simulink model "Teste_sem_maquina_sincrona"  (R2016a)
settings: Solver=VariableStepAuto  StartTime=0.0  StopTime=0.01  RelTol=1e-3
undefined symbols (not defined in the file or in its folder): D1, Delta, Ts
libraries: powerlib x42, simulink x4, simulink_extras x4, electricdrivelib x1, powerlib_meascontrol x1
settings Model: Creator=Joao  LastModifiedBy=Joao

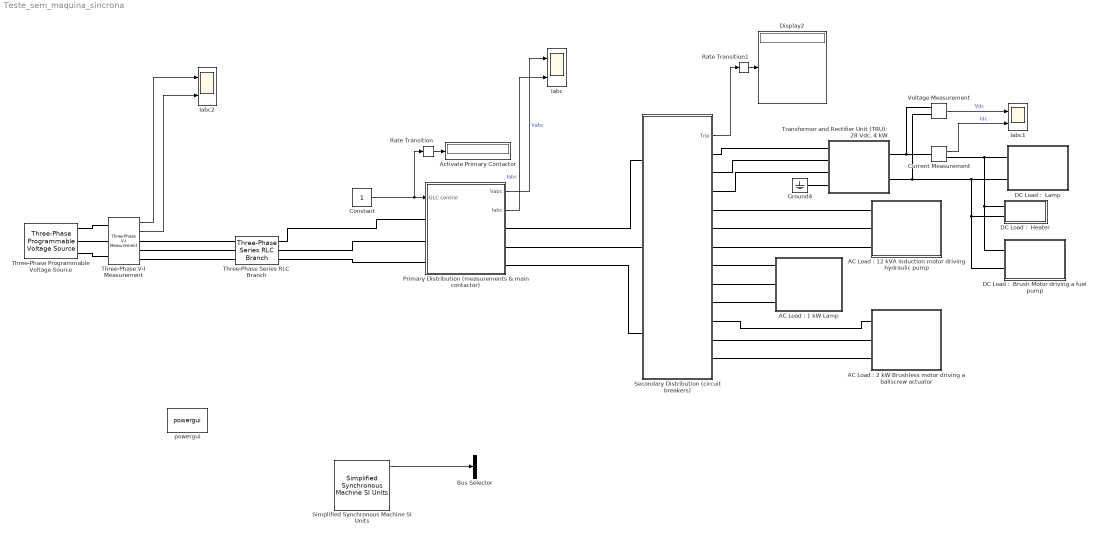
== system Teste_sem_maquina_sincrona ==
  "AC Load : 1 kW Lamp" : Subsystem
      mask Display: image(imread('power_aircraft_distribution_ACLamp.jpg','jpg'))
  "AC Load : 12 kVA induction motor driving hydraulic pump" : Subsystem
      mask Display: image(imread('power_aircraft_distribution_EnginePump.jpg','jpg'))
  "AC Load : 2 kW Brushless motor driving a ballscrew actuator" : Subsystem
      mask Display: image(imread('power_aircraft_distribution_ballscrew.jpg','jpg'))
  Activate Primary Contactor : Display
      settings: SampleTime=1e-2
  Bus Selector : BusSelector  OutputSignals=signal1,signal2
  Constant : Constant
  Current Measurement : powerlib/Measurements/Current Measurement  PhasorSimulation=off  OutputType=Complex  PSBequivalent=0
  "DC Load :  Brush Motor driving a fuel pump" : Subsystem
      mask Display: image(imread('power_aircraft_distribution_FuelPump.jpg','jpg'))
  "DC Load :  Heater" : Subsystem
      mask Display: image(imread('power_aircraft_distribution_heater.jpg','jpg'))
  "DC Load :  Lamp" : Subsystem
      mask Display: image(imread('power_aircraft_distribution_DCLamp.jpg','jpg'))
  Display2 : Display
      settings: SampleTime=1e-2
  Ground4 : powerlib/Elements/Ground  LConnTagsString=a
  Iabc : Scope  NumInputPorts=2
  Iabc1 : Scope  NumInputPorts=2
  Iabc2 : Scope  NumInputPorts=2
  Primary Distribution (measurements & main contactor) : Subsystem
  Rate Transition : RateTransition  OutPortSampleTimeOpt=Inherit  OutPortSampleTime=Ts
  Rate Transition1 : RateTransition  OutPortSampleTimeOpt=Inherit  OutPortSampleTime=Ts
  Secondary Distribution (circuit breakers) : Subsystem  mask{FuseA=25, FuseB=200, FuseC=5, FuseD=30}
      mask prompts: FuseA "Breaker  TRU (Amps RMS)"; FuseB "Breaker AC motor (Amps RMS)"; FuseC "Breaker Lamp (Amps RMS)"; FuseD "Breaker Brushless (Amps RMS)"
  Simplified Synchronous Machine SI Units : powerlib/Machines/Simplified Synchronous Machine SI Units  ConnectionType=3-wire Y  MechanicalLoad=Mechanical power Pm  MeasurementBus=off  NominalParameters=[187e6 13800 60]  Mechanical=[3.895e6 0 20]  InternalRL="[0.0204  0.8104e-3]"  InitialConditions="[ 0,0   0,0,0   0,0,0 ]"  Units=1  LoadFlowParameters=[1,0,0,0,0]  TsPowergui=0  TsBlock=-1  BusType=PV  Pref=0  Qref=0  Qmin=-inf  Qmax=+inf  PLF=0  QLF=0
  Three-Phase Programmable Voltage Source : powerlib/Electrical Sources/Three-Phase Programmable Voltage Source  PositiveSequence="[115*sqrt(3)  0 400]"  VariationEntity=None  VariationType=Table of time-amplitude pairs  VariationTypeAlt=Step  VariationStep=0.5  VariationRate=10  VariationMagnitude=0.3  VariationFrequency=2  VariationTiming=[1 2]  VariationPhaseA=off  Amplitudes=[1 0.8 1.2 1.0]  TimeValues=[0 0.1 0.15 0.2]  HarmonicGeneration=off  HarmonicA=[3 0.2 -25 0]  HarmonicB=[2 0.15 35 2]  Timing="[0.05  3]"  BusType=swing  Pref=0  Qref=0  Qmin=-inf  Qmax=inf
  Three-Phase Series RLC Branch : powerlib/Elements/Three-Phase Series RLC Branch  LConnTagsString=A|B|C  RConnTagsString=A|B|C  BranchType=RL  Resistance=0.2  Inductance=8e-4  Capacitance=0  Measurements=None
  Three-Phase V-I Measurement : powerlib/Measurements/Three-Phase V-I Measurement  VoltageMeasurement=phase-to-ground  SetLabelV=off  LabelV=Vabc  Vpu=off  VpuLL=off  CurrentMeasurement=yes  SetLabelI=off  LabelI=Iabc  Ipu=off  Pbase=100e6  Vbase=500e3  OutputType=Complex  PhasorSimulation=off  PSBequivalent=0
  "Transformer and Rectifier Unit (TRU): 28 Vdc, 4 kW" : Subsystem
      mask Display: image(imread('power_aircraft_distribution_TRU.jpg','jpg'))
  Voltage Measurement : powerlib/Measurements/Voltage Measurement  PhasorSimulation=off  OutputType=Complex  PSBequivalent=0
  powergui : powerlib/powergui  Priority=1  SimulationMode=Discrete  SolverType=Tustin/Backward Euler (TBE)  SampleTime=1e-7  frequency=60  SPID=off  DisableSnubberDevices=off  DisableRonSwitches=off  DisableVfSwitches=off  SwTol=0  DisplayEquations=off  Interpol=off  ExternalGateDelay=off  methode=off  Ts=10  FunctionMessages=off  echomessages=off  HookPort=off  EnableUseOfTLC=off  x0status=blocks  frequencyindice=0  Pbase=100e6  ErrMax=1e-4  Iterations=50  UnitsV=kV  UnitsW=MW  buscounter=0  RestoreLinks=warning  ResistiveCurrentMeasurement=off  Frange=[0:2:500]  Ylog=off  Xlog=on  ShowGrid=off  save=off  variable=ZData  structure=0  ZoomFFT=off  StartTime=0.0  cycles=1  DisplayStyle=1  fundamental=60  FreqAxis=off  MaxFrequency=1000  frequencyindicesteady=1  RmsSteady=1  display=off
  wires:
  Constant/1 -> Rate Transition/1, Primary Distribution (measurements & main contactor)/1(GLC control)
  Secondary Distribution (circuit breakers)/1(Trip) -> Rate Transition1/1
  Current Measurement/1 -> Iabc1/2  "Idc"
  Voltage Measurement/1 -> Iabc1/1  "Vdc"
  Rate Transition/1 -> Activate Primary Contactor/1
  Rate Transition1/1 -> Display2/1
  Three-Phase V-I Measurement/1 -> Iabc2/1
  Three-Phase V-I Measurement/2 -> Iabc2/2
  Primary Distribution (measurements & main contactor)/1(Vabc) -> Iabc/1  "Vabc"
  Primary Distribution (measurements & main contactor)/2(Iabc) -> Iabc/2  "Iabc"
  Simplified Synchronous Machine SI Units/1 -> Bus Selector/1
  connections:
  Current Measurement/RConn1 -- "DC Load :  Lamp"/LConn1 -- "DC Load :  Heater"/LConn1 -- "DC Load :  Brush Motor driving a fuel pump"/LConn1
  Voltage Measurement/LConn1 -- "Transformer and Rectifier Unit (TRU): 28 Vdc, 4 kW"/RConn1 -- Current Measurement/LConn1
  "DC Load :  Lamp"/LConn2 -- Voltage Measurement/LConn2 -- "Transformer and Rectifier Unit (TRU): 28 Vdc, 4 kW"/RConn2 -- "DC Load :  Heater"/LConn2 -- "DC Load :  Brush Motor driving a fuel pump"/LConn2
  Secondary Distribution (circuit breakers)/RConn8 -- "AC Load : 1 kW Lamp"/LConn2
  Secondary Distribution (circuit breakers)/RConn10 -- "AC Load : 2 kW Brushless motor driving a ballscrew actuator"/LConn1
  Secondary Distribution (circuit breakers)/RConn4 -- "AC Load : 12 kVA induction motor driving hydraulic pump"/LConn1
  Secondary Distribution (circuit breakers)/RConn12 -- "AC Load : 2 kW Brushless motor driving a ballscrew actuator"/LConn3
  Secondary Distribution (circuit breakers)/RConn11 -- "AC Load : 2 kW Brushless motor driving a ballscrew actuator"/LConn2
  Ground4/LConn1 -- "Transformer and Rectifier Unit (TRU): 28 Vdc, 4 kW"/LConn4
  Secondary Distribution (circuit breakers)/LConn2 -- Primary Distribution (measurements & main contactor)/RConn2
  Secondary Distribution (circuit breakers)/LConn3 -- Primary Distribution (measurements & main contactor)/RConn3
  Secondary Distribution (circuit breakers)/RConn6 -- "AC Load : 12 kVA induction motor driving hydraulic pump"/LConn3
  Secondary Distribution (circuit breakers)/RConn5 -- "AC Load : 12 kVA induction motor driving hydraulic pump"/LConn2
  Secondary Distribution (circuit breakers)/RConn7 -- "AC Load : 1 kW Lamp"/LConn1
  Secondary Distribution (circuit breakers)/RConn2 -- "Transformer and Rectifier Unit (TRU): 28 Vdc, 4 kW"/LConn2
  Secondary Distribution (circuit breakers)/RConn9 -- "AC Load : 1 kW Lamp"/LConn3
  Secondary Distribution (circuit breakers)/RConn1 -- "Transformer and Rectifier Unit (TRU): 28 Vdc, 4 kW"/LConn1
  Primary Distribution (measurements & main contactor)/RConn1 -- Secondary Distribution (circuit breakers)/LConn1
  Secondary Distribution (circuit breakers)/RConn3 -- "Transformer and Rectifier Unit (TRU): 28 Vdc, 4 kW"/LConn3
  Primary Distribution (measurements & main contactor)/LConn1 -- Three-Phase Series RLC Branch/RConn1
  Primary Distribution (measurements & main contactor)/LConn2 -- Three-Phase Series RLC Branch/RConn2
  Primary Distribution (measurements & main contactor)/LConn3 -- Three-Phase Series RLC Branch/RConn3
  Three-Phase Programmable Voltage Source/RConn1 -- Three-Phase V-I Measurement/LConn1
  Three-Phase Programmable Voltage Source/RConn2 -- Three-Phase V-I Measurement/LConn2
  Three-Phase Programmable Voltage Source/RConn3 -- Three-Phase V-I Measurement/LConn3
  Three-Phase V-I Measurement/RConn1 -- Three-Phase Series RLC Branch/LConn1
  Three-Phase V-I Measurement/RConn2 -- Three-Phase Series RLC Branch/LConn2
  Three-Phase V-I Measurement/RConn3 -- Three-Phase Series RLC Branch/LConn3

== system Teste_sem_maquina_sincrona/AC Load : 1 kW Lamp ==
  note: AC Load
  Lamp 1000 Watts : powerlib/Elements/Three-Phase Series RLC Load  LConnTagsString=A|B|C  Configuration=Y (grounded)  NominalVoltage=200  Vabc=[1e3 1e3 1e3]  Vabcp=[1e3 1e3 1e3]  NominalFrequency=400  UnbalancedPower=off  ActivePower=1000  InductivePower=0  CapacitivePower=0  Pabc=[10e3 9e3 11e3]  QLabc=[100 90 110]  QCabc=[100 90 110]  Pabcp=[10e3 9e3 11e3]  QLabcp=[100 90 110]  QCabcp=[100 90 110]  Measurements=None  LoadType=constant Z
  A : PMIOPort  Port=1  Side=Left
  B : PMIOPort  Port=2  Side=Left
  C : PMIOPort  Port=3  Side=Left
  connections:
  A/RConn1 -- Lamp 1000 Watts/LConn1
  B/RConn1 -- Lamp 1000 Watts/LConn2
  C/RConn1 -- Lamp 1000 Watts/LConn3

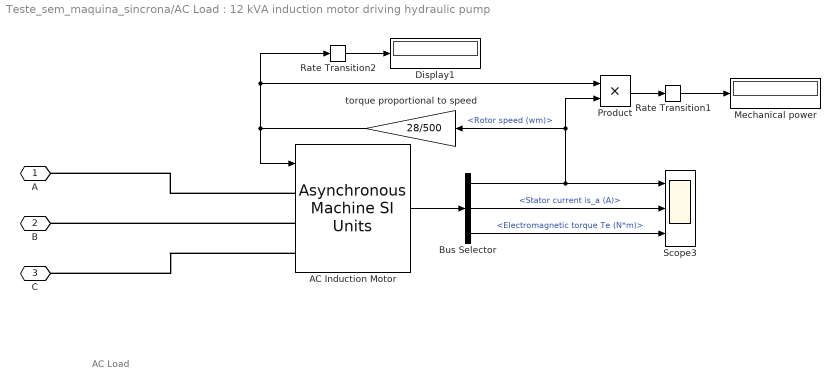
== system Teste_sem_maquina_sincrona/AC Load : 12 kVA induction motor driving hydraulic pump ==
  note: AC Load
  AC Induction Motor : powerlib/Machines/Asynchronous Machine SI Units  RotorType=Squirrel-cage  PresetModel=No  MechanicalLoad=Torque Tm  ShowDetailedParameters=on  ReferenceFrame=Rotor  Units=SI  MeasurementBus=off  NominalParameters=[12e3 200 400]  Stator=[0.2761 0.002191/10]  Rotor=[0.16 0.002191/10]  Cage1=[ 0.022 0.226/377]  Cage2=[ 0.022 0.226/377]  Lm=0.07614  Mechanical=[0.01 0 8]  PolePairs=8  InitialConditions=[1,0 0,0,0 0,0,0]  SimulateSaturation=off  Saturation=[14.03593122, 27.81365428, 53.79336849, 72.68890987, 97.98006896, 148.6815601, 215.7428561, 302.9841135, 428.7778367 ; 230, 322, 414, 460, 506, 552, 598, 644, 690]  LoadFlowParameters=0  TsPowergui=0  TsBlock=-1  IterativeModel=Trapezoidal non iterative  IterativeDiscreteModel=Trapezoidal non iterative  Pmec=0
  Bus Selector : BusSelector  OutputSignals=Mechanical.Rotor speed (wm),Stator measurements.Stator current is_a (A),Mechanical.Electromagnetic torque Te (N*m)
  Display1 : Display
      settings: SampleTime=1e-2
  Mechanical power : Display
      settings: SampleTime=1e-2
  Product : Product  RndMeth=Zero
  Rate Transition1 : RateTransition  OutPortSampleTimeOpt=Inherit  OutPortSampleTime=Ts
  Rate Transition2 : RateTransition  OutPortSampleTimeOpt=Inherit  OutPortSampleTime=Ts
  Scope3 : Scope  NumInputPorts=3
  torque proportional to speed : Gain  Gain=28/500
  A : PMIOPort  Port=1  Side=Left
  B : PMIOPort  Port=2  Side=Left
  C : PMIOPort  Port=3  Side=Left
  wires:
  AC Induction Motor/1 -> Bus Selector/1
  Bus Selector/1 -> Scope3/1, torque proportional to speed/1, Product/2  "<Rotor speed (wm)>"
  torque proportional to speed/1 -> AC Induction Motor/1, Product/1, Rate Transition2/1
  Product/1 -> Rate Transition1/1
  Bus Selector/2 -> Scope3/2  "<Stator current is_a (A)>"
  Bus Selector/3 -> Scope3/3  "<Electromagnetic torque Te (N*m)>"
  Rate Transition1/1 -> Mechanical power/1
  Rate Transition2/1 -> Display1/1
  connections:
  AC Induction Motor/LConn2 -- B/RConn1
  AC Induction Motor/LConn1 -- A/RConn1
  AC Induction Motor/LConn3 -- C/RConn1

== system Teste_sem_maquina_sincrona/AC Load : 2 kW Brushless motor driving a ballscrew actuator ==
  note: AC Load
  Gain : Gain  Gain=0.2
  Line inductor : powerlib/Elements/Three-Phase Series RLC Branch  LConnTagsString=A|B|C  RConnTagsString=A|B|C  BranchType=L  Resistance=[]  Inductance=1e-3  Capacitance=[]  Measurements=None
  PM Synchronous Motor Drive : electricdrivelib/AC drives/PM Synchronous Motor Drive  showMaskWarnings=on  AverageValue=on  MechanicalLoad=Torque Tm  driveType=AC6  outputBusMode=Multiple output buses  baseSampleTime=1e-07
      link override Braking chopper: capacitance=2000e-6  Setx0=on  InitialVoltage=300  Rbrake=8  frequency=4000  activationVoltage=290  shutdownVoltage=280
      link override VECT: freq_max=20e3  Ts_vect=50e-6  h=0.1  nb_p=4  lambda=0.175
  Scope : Scope  NumInputPorts=4
  Speed : powerlib_meascontrol/Pulse & Signal Generators/Stair Generator  t=[0 1.4 1.9 2.4 3]  e=[0 500 0 -500 0]  Ts=Ts
  demux : Subsystem
  A : PMIOPort  Port=1  Side=Left
  B : PMIOPort  Port=2  Side=Left
  C : PMIOPort  Port=3  Side=Left
  wires:
  Speed/1 -> PM Synchronous Motor Drive/1
  Gain/1 -> PM Synchronous Motor Drive/2
  demux/1(i_a) -> Scope/1  "Stator current"
  demux/2(speed) -> Scope/2  "Rotor speed"
  demux/3(Tem) -> Scope/3  "Electromagnetic Torque"
  demux/4(v_dc) -> Scope/4  "DC bus voltage"
  PM Synchronous Motor Drive/4 -> Gain/1
  PM Synchronous Motor Drive/1 -> demux/1(motor)
  PM Synchronous Motor Drive/2 -> demux/2(Conv.)
  PM Synchronous Motor Drive/3 -> demux/3(Ctrl)
  connections:
  PM Synchronous Motor Drive/LConn3 -- Line inductor/RConn3
  PM Synchronous Motor Drive/LConn2 -- Line inductor/RConn2
  PM Synchronous Motor Drive/LConn1 -- Line inductor/RConn1
  Line inductor/LConn3 -- C/RConn1
  Line inductor/LConn2 -- B/RConn1
  Line inductor/LConn1 -- A/RConn1

== system Teste_sem_maquina_sincrona/DC Load :  Brush Motor driving a fuel pump ==
  note: DC Load
  Bus Selector : BusSelector  OutputSignals=Speed wm (rad/s),Armature current ia (A),Electrical torque Te (n m)
  DC Machine : powerlib/Machines/DC Machine  PresetModel=No  MechanicalLoad=Torque TL  FieldType=Wound  ShowDetailedParameters=on  MeasurementBus=off  RLa=[ .35 0.0001]  RLf="[ 240  12]"  Laf=1  MachineConstant=Torque constant (N.m/A)  Ke=1.8  Kt=1.8  J=0.0005  Bm=0  Tf=0  w0=0  Ifinit=0  TsPowergui=0  TsBlock=-1
  Gain : Gain  Gain=1.5/200
  Scope3 : Scope  NumInputPorts=3
  + : PMIOPort  Port=1  Side=Left
  - : PMIOPort  Port=2  Side=Left
  wires:
  Gain/1 -> DC Machine/1
  DC Machine/1 -> Bus Selector/1
  Bus Selector/1 -> Scope3/1, Gain/1  "<Speed wm (rad/s)>"
  Bus Selector/2 -> Scope3/2  "<Armature current ia (A)>"
  Bus Selector/3 -> Scope3/3  "<Electrical torque Te (n m)>"
  connections:
  -/RConn1 -- DC Machine/RConn1 -- DC Machine/RConn2
  +/RConn1 -- DC Machine/LConn1 -- DC Machine/LConn2

== system Teste_sem_maquina_sincrona/DC Load :  Heater ==
  note: DC Load
  Series RLC Branch3 : powerlib/Elements/Series RLC Branch  LConnTagsString=__new0  RConnTagsString=__new0  BranchType=R  Resistance=1  Inductance=[]  SetiL0=off  InitialCurrent=0  Capacitance=[]  Setx0=off  InitialVoltage=0  Measurements=Branch voltage and current
  + : PMIOPort  Port=1  Side=Left
  - : PMIOPort  Port=2  Side=Left
  connections:
  -/RConn1 -- Series RLC Branch3/RConn1
  +/RConn1 -- Series RLC Branch3/LConn1

== system Teste_sem_maquina_sincrona/DC Load :  Lamp ==
  note: DC Load
  Series RLC Branch3 : powerlib/Elements/Series RLC Branch  LConnTagsString=__new0  RConnTagsString=__new0  BranchType=R  Resistance=1  Inductance=[]  SetiL0=off  InitialCurrent=0  Capacitance=[]  Setx0=off  InitialVoltage=0  Measurements=Branch voltage and current
  + : PMIOPort  Port=1  Side=Left
  - : PMIOPort  Port=2  Side=Left
  connections:
  +/RConn1 -- Series RLC Branch3/LConn1
  -/RConn1 -- Series RLC Branch3/RConn1

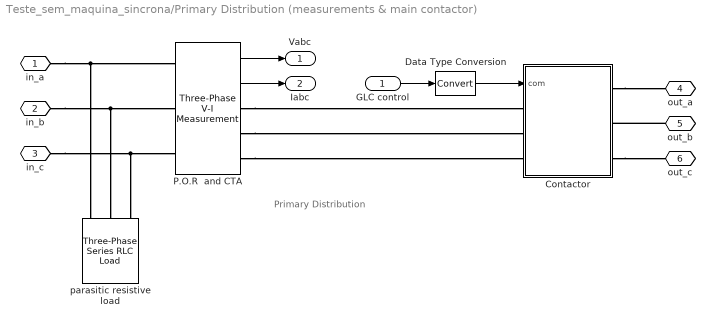
== system Teste_sem_maquina_sincrona/Primary Distribution (measurements & main contactor) ==
  note: Primary Distribution
  GLC control : Inport
  Contactor : Subsystem
  Data Type Conversion : DataTypeConversion
  P.O.R  and CTA : powerlib/Measurements/Three-Phase V-I Measurement  VoltageMeasurement=phase-to-phase  SetLabelV=off  LabelV=Vabc  Vpu=off  VpuLL=off  CurrentMeasurement=yes  SetLabelI=off  LabelI=Iabc  Ipu=off  Pbase=100e6  Vbase=500e3  OutputType=Complex  PhasorSimulation=off  PSBequivalent=0
  parasitic resistive load : powerlib/Elements/Three-Phase Series RLC Load  LConnTagsString=A|B|C  Configuration=Y (grounded)  NominalVoltage=200  Vabc=[1e3 1e3 1e3]  Vabcp=[1e3 1e3 1e3]  NominalFrequency=400  UnbalancedPower=off  ActivePower=5000  InductivePower=0  CapacitivePower=0  Pabc=[10e3 9e3 11e3]  QLabc=[100 90 110]  QCabc=[100 90 110]  Pabcp=[10e3 9e3 11e3]  QLabcp=[100 90 110]  QCabcp=[100 90 110]  Measurements=None  LoadType=constant Z
  in_a : PMIOPort  Port=1  Side=Left
  in_b : PMIOPort  Port=2  Side=Left
  in_c : PMIOPort  Port=3  Side=Left
  out_a : PMIOPort  Port=4  Side=Right
  out_b : PMIOPort  Port=5  Side=Right
  out_c : PMIOPort  Port=6  Side=Right
  Vabc : Outport
  Iabc : Outport  Port=2
  wires:
  GLC control/1 -> Data Type Conversion/1
  P.O.R  and CTA/1 -> Vabc/1
  P.O.R  and CTA/2 -> Iabc/1
  Data Type Conversion/1 -> Contactor/1(com)
  connections:
  in_a/RConn1 -- P.O.R  and CTA/LConn1 -- parasitic resistive load/LConn1
  in_b/RConn1 -- P.O.R  and CTA/LConn2 -- parasitic resistive load/LConn2
  in_c/RConn1 -- P.O.R  and CTA/LConn3 -- parasitic resistive load/LConn3
  P.O.R  and CTA/RConn1 -- Contactor/LConn1
  P.O.R  and CTA/RConn2 -- Contactor/LConn2
  P.O.R  and CTA/RConn3 -- Contactor/LConn3
  Contactor/RConn1 -- out_a/RConn1
  out_b/RConn1 -- Contactor/RConn2
  Contactor/RConn3 -- out_c/RConn1

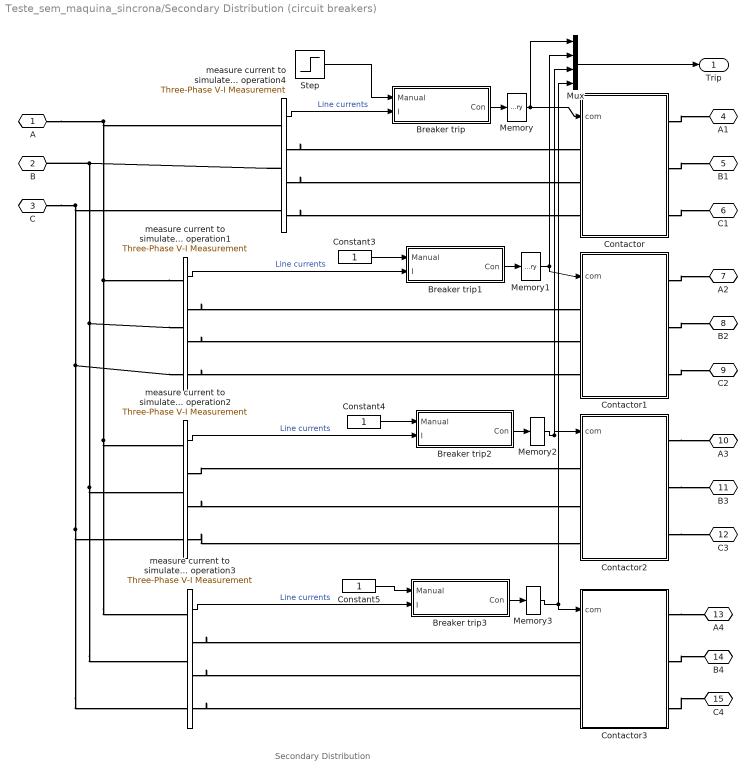
== system Teste_sem_maquina_sincrona/Secondary Distribution (circuit breakers) ==
  note: Secondary Distribution
  Breaker trip : Subsystem
  Breaker trip1 : Subsystem
  Breaker trip2 : Subsystem
  Breaker trip3 : Subsystem
  Constant3 : Constant  OutDataTypeStr=boolean
  Constant4 : Constant  OutDataTypeStr=boolean
  Constant5 : Constant  OutDataTypeStr=boolean
  Contactor : Subsystem
  Contactor1 : Subsystem
  Contactor2 : Subsystem
  Contactor3 : Subsystem
  Memory{,1..3} (4 alike) : Memory
  Mux : Mux
  Step : Step  Time=3.5  Before=1  After=0  SampleTime=0
  measure current to simulate fuse operation{1..4} (4 alike) : powerlib/Measurements/Three-Phase V-I Measurement  VoltageMeasurement=no  SetLabelV=off  LabelV=Vabc  Vpu=off  VpuLL=off  CurrentMeasurement=yes  SetLabelI=off  LabelI=Iabc  Ipu=off  Pbase=100e6  Vbase=500e3  OutputType=Complex  PhasorSimulation=off  PSBequivalent=0
  A : PMIOPort  Port=1  Side=Left
  B : PMIOPort  Port=2  Side=Left
  C : PMIOPort  Port=3  Side=Left
  A1 : PMIOPort  Port=4  Side=Right
  B1 : PMIOPort  Port=5  Side=Right
  C1 : PMIOPort  Port=6  Side=Right
  A2 : PMIOPort  Port=7  Side=Right
  B2 : PMIOPort  Port=8  Side=Right
  C2 : PMIOPort  Port=9  Side=Right
  A3 : PMIOPort  Port=10  Side=Right
  B3 : PMIOPort  Port=11  Side=Right
  C3 : PMIOPort  Port=12  Side=Right
  A4 : PMIOPort  Port=13  Side=Right
  B4 : PMIOPort  Port=14  Side=Right
  C4 : PMIOPort  Port=15  Side=Right
  Trip : Outport
  wires:
  Constant3/1 -> Breaker trip1/1(Manual)
  Step/1 -> Breaker trip/1(Manual)
  Memory3/1 -> Contactor3/1(com), Mux/4
  Memory2/1 -> Contactor2/1(com), Mux/3
  Breaker trip1/1(Con) -> Memory1/1
  Memory/1 -> Contactor/1(com), Mux/1
  Memory1/1 -> Contactor1/1(com), Mux/2
  Mux/1 -> Trip/1
  Breaker trip2/1(Con) -> Memory2/1
  Breaker trip3/1(Con) -> Memory3/1
  Constant4/1 -> Breaker trip2/1(Manual)
  Constant5/1 -> Breaker trip3/1(Manual)
  measure current to simulate fuse operation3/1 -> Breaker trip3/2(I)  "Line currents"
  measure current to simulate fuse operation2/1 -> Breaker trip2/2(I)  "Line currents"
  measure current to simulate fuse operation1/1 -> Breaker trip1/2(I)  "Line currents"
  Breaker trip/1(Con) -> Memory/1
  measure current to simulate fuse operation4/1 -> Breaker trip/2(I)  "Line currents"
  connections:
  measure current to simulate fuse operation3/RConn3 -- Contactor3/LConn3
  measure current to simulate fuse operation3/RConn2 -- Contactor3/LConn2
  measure current to simulate fuse operation3/RConn1 -- Contactor3/LConn1
  Contactor3/RConn3 -- C4/RConn1
  Contactor3/RConn2 -- B4/RConn1
  Contactor3/RConn1 -- A4/RConn1
  measure current to simulate fuse operation2/RConn3 -- Contactor2/LConn3
  measure current to simulate fuse operation2/RConn2 -- Contactor2/LConn2
  measure current to simulate fuse operation2/RConn1 -- Contactor2/LConn1
  Contactor2/RConn3 -- C3/RConn1
  Contactor2/RConn2 -- B3/RConn1
  Contactor2/RConn1 -- A3/RConn1
  measure current to simulate fuse operation1/RConn3 -- Contactor1/LConn3
  measure current to simulate fuse operation1/RConn2 -- Contactor1/LConn2
  measure current to simulate fuse operation1/RConn1 -- Contactor1/LConn1
  Contactor1/RConn3 -- C2/RConn1
  Contactor1/RConn2 -- B2/RConn1
  Contactor1/RConn1 -- A2/RConn1
  measure current to simulate fuse operation4/RConn3 -- Contactor/LConn3
  measure current to simulate fuse operation4/RConn2 -- Contactor/LConn2
  measure current to simulate fuse operation4/RConn1 -- Contactor/LConn1
  Contactor/RConn3 -- C1/RConn1
  Contactor/RConn2 -- B1/RConn1
  Contactor/RConn1 -- A1/RConn1
  measure current to simulate fuse operation1/LConn3 -- measure current to simulate fuse operation4/LConn3 -- C/RConn1 -- measure current to simulate fuse operation2/LConn3 -- measure current to simulate fuse operation3/LConn3
  measure current to simulate fuse operation1/LConn2 -- measure current to simulate fuse operation2/LConn2 -- measure current to simulate fuse operation3/LConn2 -- B/RConn1 -- measure current to simulate fuse operation4/LConn2
  measure current to simulate fuse operation1/LConn1 -- measure current to simulate fuse operation2/LConn1 -- measure current to simulate fuse operation3/LConn1 -- measure current to simulate fuse operation4/LConn1 -- A/RConn1

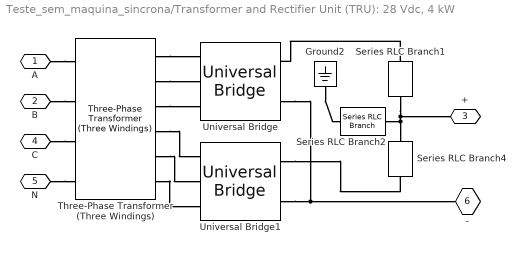
== system Teste_sem_maquina_sincrona/Transformer and Rectifier Unit (TRU): 28 Vdc, 4 kW ==
  Ground2 : powerlib/Elements/Ground  LConnTagsString=a
  Series RLC Branch1 : powerlib/Elements/Series RLC Branch  LConnTagsString=__new0  RConnTagsString=__new0  BranchType=L  Resistance=[]  Inductance=2e-3  SetiL0=on  InitialCurrent=0  Capacitance=[]  Setx0=off  InitialVoltage=0  Measurements=Branch voltage and current
  Series RLC Branch2 : powerlib/Elements/Series RLC Branch  LConnTagsString=__new0  RConnTagsString=__new0  BranchType=C  Resistance=[]  Inductance=[]  SetiL0=off  InitialCurrent=0  Capacitance=1e-6  Setx0=off  InitialVoltage=0  Measurements=None
  Series RLC Branch4 : powerlib/Elements/Series RLC Branch  LConnTagsString=__new0  RConnTagsString=__new0  BranchType=L  Resistance=[]  Inductance=2e-3  SetiL0=off  InitialCurrent=0  Capacitance=[]  Setx0=off  InitialVoltage=0  Measurements=Branch voltage and current
  Three-Phase Transformer (Three Windings) : powerlib/Elements/Three-Phase Transformer (Three Windings)  Winding1Connection=Yn  Winding2Connection=Delta (D1)  Winding3Connection=Delta (D1)  CoreType=Three single-phase transformers  SetSaturation=off  Hysteresis=off  DataFile='hysteresis'  SetInitialFlux=off  Measurements=None  UNITS=pu  NominalPower=[ 4200 , 600 ]  Winding1=[ 200 , 0.0002 , 0 ]  Winding2=[ 22 , 0.0002 , 0 ]  Winding3=[ 22 , 0.0002 , 0]  Rm=500  Lm=500*10  L0=0.5  Saturation=[ 0,0 ; 0.0024,1.2 ; 1.0,1.52 ]  InitialFluxes=[0.8 -0.8 0.7]  MoreParameters=off  BreakLoop=off  DataType=off  TransfoNumber=0
  Universal Bridge : powerlib/Power Electronics/Universal Bridge  Arms=3  SnubberResistance=1e3  SnubberCapacitance=1e-6  Device=Diodes  Ron=1e-3  Lon=0  ForwardVoltages="[  0  0  ]"  ForwardVoltage=0.8  GTOparameters=[ 10e-6 , 20e-6 ]  IGBTparameters=[ 1e-6 , 2e-6 ]  Measurements=None  Measurements_2=None  converterType=Rectifier
  Universal Bridge1 : powerlib/Power Electronics/Universal Bridge  Arms=3  SnubberResistance=1e3  SnubberCapacitance=1e-6  Device=Diodes  Ron=1e-3  Lon=0  ForwardVoltages="[  0  0  ]"  ForwardVoltage=0.8  GTOparameters=[ 10e-6 , 20e-6 ]  IGBTparameters=[ 1e-6 , 2e-6 ]  Measurements=None  Measurements_2=None  converterType=Rectifier
  A : PMIOPort  Port=1  Side=Left
  B : PMIOPort  Port=2  Side=Left
  + : PMIOPort  Port=3  Side=Right
  C : PMIOPort  Port=4  Side=Left
  N : PMIOPort  Port=5  Side=Left
  - : PMIOPort  Port=6  Side=Right
  connections:
  Ground2/LConn1 -- Series RLC Branch2/RConn1
  Universal Bridge/RConn2 -- Universal Bridge1/RConn2 -- -/RConn1
  Three-Phase Transformer (Three Windings)/RConn1 -- Universal Bridge/LConn1
  Three-Phase Transformer (Three Windings)/RConn2 -- Universal Bridge/LConn2
  Three-Phase Transformer (Three Windings)/RConn3 -- Universal Bridge/LConn3
  A/RConn1 -- Three-Phase Transformer (Three Windings)/LConn1
  B/RConn1 -- Three-Phase Transformer (Three Windings)/LConn2
  C/RConn1 -- Three-Phase Transformer (Three Windings)/LConn3
  N/RConn1 -- Three-Phase Transformer (Three Windings)/LConn4
  Series RLC Branch1/LConn1 -- Universal Bridge/RConn1
  Series RLC Branch2/LConn1 -- Series RLC Branch1/RConn1 -- +/RConn1 -- Series RLC Branch4/LConn1
  Three-Phase Transformer (Three Windings)/RConn4 -- Universal Bridge1/LConn1
  Three-Phase Transformer (Three Windings)/RConn5 -- Universal Bridge1/LConn2
  Three-Phase Transformer (Three Windings)/RConn6 -- Universal Bridge1/LConn3
  Universal Bridge1/RConn1 -- Series RLC Branch4/RConn1

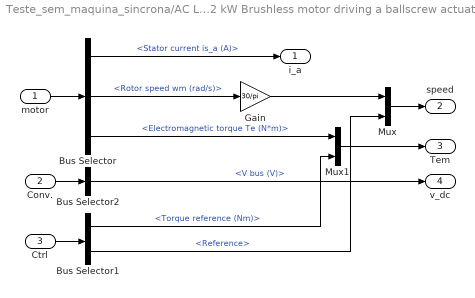
== system Teste_sem_maquina_sincrona/AC Load : 2 kW Brushless motor driving a ballscrew actuator/demux ==
  motor : Inport
  Conv. : Inport  Port=2
  Ctrl : Inport  Port=3
  Bus Selector : BusSelector  OutputSignals=Stator current is_a (A),Rotor speed wm (rad/s),Electromagnetic torque Te (N*m)
  Bus Selector1 : BusSelector  OutputSignals=Torque reference (Nm),Reference
  Bus Selector2 : BusSelector  OutputSignals=V bus (V)
  Gain : Gain  Gain=30/pi  SaturateOnIntegerOverflow=on  OutDataTypeStr=Inherit: Same as input  ParamDataTypeStr=Inherit: Same as input
  Mux : Mux  Inputs=2
  Mux1 : Mux  Inputs=2
  i_a : Outport
  speed : Outport  Port=2
  Tem : Outport  Port=3
  v_dc : Outport  Port=4
  wires:
  Bus Selector/2 -> Gain/1  "<Rotor speed wm (rad/s)>"
  Bus Selector2/1 -> v_dc/1  "<V bus (V)>"
  Conv./1 -> Bus Selector2/1
  Ctrl/1 -> Bus Selector1/1
  Bus Selector1/1 -> Mux1/2  "<Torque reference (Nm)>"
  Bus Selector1/2 -> Mux/2  "<Reference>"
  Gain/1 -> Mux/1
  Bus Selector/1 -> i_a/1  "<Stator current is_a (A)>"
  Bus Selector/3 -> Mux1/1  "<Electromagnetic torque Te (N*m)>"
  Mux1/1 -> Tem/1
  Mux/1 -> speed/1
  motor/1 -> Bus Selector/1

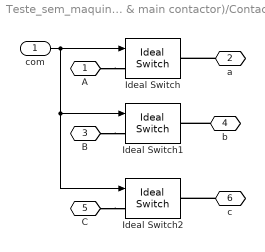
== system Teste_sem_maquina_sincrona/Primary Distribution (measurements & main contactor)/Contactor ==
  com : Inport
  Ideal Switch : powerlib/Power Electronics/Ideal Switch  Ron=0.001  Lon=0  IC=0  Rs=1e3  Cs=inf  Measurements=off
  Ideal Switch1 : powerlib/Power Electronics/Ideal Switch  Ron=0.001  Lon=0  IC=0  Rs=1e3  Cs=inf  Measurements=off
  Ideal Switch2 : powerlib/Power Electronics/Ideal Switch  Ron=0.001  Lon=0  IC=0  Rs=1e3  Cs=inf  Measurements=off
  A : PMIOPort  Port=1  Side=Left
  a : PMIOPort  Port=2  Side=Right
  B : PMIOPort  Port=3  Side=Left
  b : PMIOPort  Port=4  Side=Right
  C : PMIOPort  Port=5  Side=Left
  c : PMIOPort  Port=6  Side=Right
  wires:
  com/1 -> Ideal Switch1/1, Ideal Switch2/1, Ideal Switch/1
  connections:
  c/RConn1 -- Ideal Switch2/RConn1
  C/RConn1 -- Ideal Switch2/LConn1
  b/RConn1 -- Ideal Switch1/RConn1
  B/RConn1 -- Ideal Switch1/LConn1
  a/RConn1 -- Ideal Switch/RConn1
  A/RConn1 -- Ideal Switch/LConn1

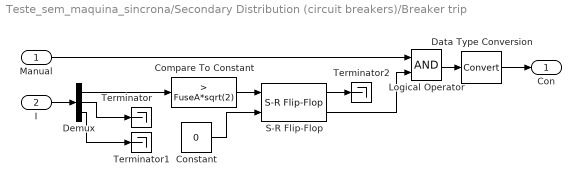
== system Teste_sem_maquina_sincrona/Secondary Distribution (circuit breakers)/Breaker trip ==
  Manual : Inport
  I : Inport  Port=2
  Compare To Constant : simulink/Logic and Bit Operations/Compare To Constant  relop=>  const=FuseA*sqrt(2)  OutDataTypeStr=boolean  ZeroCross=off
  Constant : Constant  Value=0  OutDataTypeStr=boolean
  Data Type Conversion : DataTypeConversion
  Demux : Demux  Outputs=3
  Logical Operator : Logic  AllPortsSameDT=off  OutDataTypeStr=boolean
  S-R Flip-Flop : simulink_extras/Flip Flops/S-R Flip-Flop  initial_condition=0
  Terminator : Terminator
  Terminator1 : Terminator
  Terminator2 : Terminator
  Con : Outport
  wires:
  S-R Flip-Flop/2 -> Logical Operator/2
  S-R Flip-Flop/1 -> Terminator2/1
  Constant/1 -> S-R Flip-Flop/2
  Demux/3 -> Terminator1/1
  Demux/2 -> Terminator/1
  Compare To Constant/1 -> S-R Flip-Flop/1
  Data Type Conversion/1 -> Con/1
  Manual/1 -> Logical Operator/1
  Logical Operator/1 -> Data Type Conversion/1
  Demux/1 -> Compare To Constant/1
  I/1 -> Demux/1

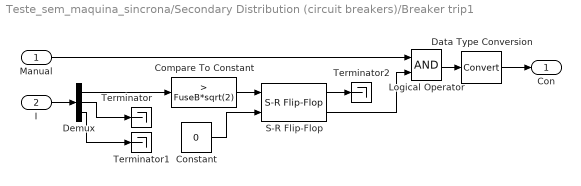
== system Teste_sem_maquina_sincrona/Secondary Distribution (circuit breakers)/Breaker trip1 ==
  Manual : Inport
  I : Inport  Port=2
  Compare To Constant : simulink/Logic and Bit Operations/Compare To Constant  relop=>  const=FuseB*sqrt(2)  OutDataTypeStr=boolean  ZeroCross=off
  Constant : Constant  Value=0  OutDataTypeStr=boolean
  Data Type Conversion : DataTypeConversion
  Demux : Demux  Outputs=3
  Logical Operator : Logic  AllPortsSameDT=off  OutDataTypeStr=boolean
  S-R Flip-Flop : simulink_extras/Flip Flops/S-R Flip-Flop  initial_condition=0
  Terminator : Terminator
  Terminator1 : Terminator
  Terminator2 : Terminator
  Con : Outport
  wires:
  I/1 -> Demux/1
  Demux/1 -> Compare To Constant/1
  Logical Operator/1 -> Data Type Conversion/1
  Manual/1 -> Logical Operator/1
  Data Type Conversion/1 -> Con/1
  Compare To Constant/1 -> S-R Flip-Flop/1
  Demux/2 -> Terminator/1
  Demux/3 -> Terminator1/1
  Constant/1 -> S-R Flip-Flop/2
  S-R Flip-Flop/1 -> Terminator2/1
  S-R Flip-Flop/2 -> Logical Operator/2

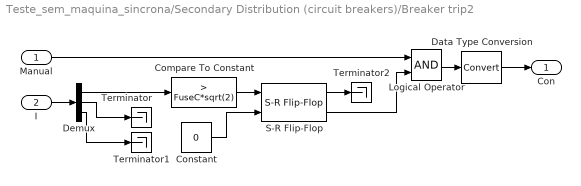
== system Teste_sem_maquina_sincrona/Secondary Distribution (circuit breakers)/Breaker trip2 ==
  Manual : Inport
  I : Inport  Port=2
  Compare To Constant : simulink/Logic and Bit Operations/Compare To Constant  relop=>  const=FuseC*sqrt(2)  OutDataTypeStr=boolean  ZeroCross=off
  Constant : Constant  Value=0  OutDataTypeStr=boolean
  Data Type Conversion : DataTypeConversion
  Demux : Demux  Outputs=3
  Logical Operator : Logic  AllPortsSameDT=off  OutDataTypeStr=boolean
  S-R Flip-Flop : simulink_extras/Flip Flops/S-R Flip-Flop  initial_condition=0
  Terminator : Terminator
  Terminator1 : Terminator
  Terminator2 : Terminator
  Con : Outport
  wires:
  S-R Flip-Flop/2 -> Logical Operator/2
  S-R Flip-Flop/1 -> Terminator2/1
  Constant/1 -> S-R Flip-Flop/2
  Demux/3 -> Terminator1/1
  Demux/2 -> Terminator/1
  Compare To Constant/1 -> S-R Flip-Flop/1
  Data Type Conversion/1 -> Con/1
  Manual/1 -> Logical Operator/1
  Logical Operator/1 -> Data Type Conversion/1
  Demux/1 -> Compare To Constant/1
  I/1 -> Demux/1

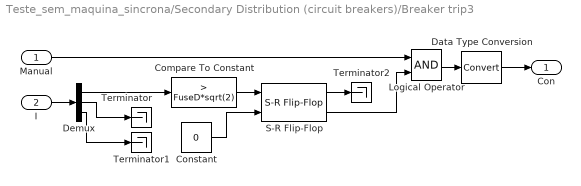
== system Teste_sem_maquina_sincrona/Secondary Distribution (circuit breakers)/Breaker trip3 ==
  Manual : Inport
  I : Inport  Port=2
  Compare To Constant : simulink/Logic and Bit Operations/Compare To Constant  relop=>  const=FuseD*sqrt(2)  OutDataTypeStr=boolean  ZeroCross=off
  Constant : Constant  Value=0  OutDataTypeStr=boolean
  Data Type Conversion : DataTypeConversion
  Demux : Demux  Outputs=3
  Logical Operator : Logic  AllPortsSameDT=off  OutDataTypeStr=boolean
  S-R Flip-Flop : simulink_extras/Flip Flops/S-R Flip-Flop  initial_condition=0
  Terminator : Terminator
  Terminator1 : Terminator
  Terminator2 : Terminator
  Con : Outport
  wires:
  I/1 -> Demux/1
  Demux/1 -> Compare To Constant/1
  Logical Operator/1 -> Data Type Conversion/1
  Manual/1 -> Logical Operator/1
  Data Type Conversion/1 -> Con/1
  Compare To Constant/1 -> S-R Flip-Flop/1
  Demux/2 -> Terminator/1
  Demux/3 -> Terminator1/1
  Constant/1 -> S-R Flip-Flop/2
  S-R Flip-Flop/1 -> Terminator2/1
  S-R Flip-Flop/2 -> Logical Operator/2

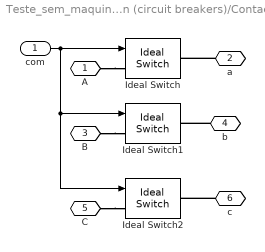
== system Teste_sem_maquina_sincrona/Secondary Distribution (circuit breakers)/Contactor ==
  com : Inport
  Ideal Switch : powerlib/Power Electronics/Ideal Switch  Ron=0.001  Lon=0  IC=0  Rs=1e3  Cs=inf  Measurements=off
  Ideal Switch1 : powerlib/Power Electronics/Ideal Switch  Ron=0.001  Lon=0  IC=0  Rs=1e3  Cs=inf  Measurements=off
  Ideal Switch2 : powerlib/Power Electronics/Ideal Switch  Ron=0.001  Lon=0  IC=0  Rs=1e3  Cs=inf  Measurements=off
  A : PMIOPort  Port=1  Side=Left
  a : PMIOPort  Port=2  Side=Right
  B : PMIOPort  Port=3  Side=Left
  b : PMIOPort  Port=4  Side=Right
  C : PMIOPort  Port=5  Side=Left
  c : PMIOPort  Port=6  Side=Right
  wires:
  com/1 -> Ideal Switch/1, Ideal Switch2/1, Ideal Switch1/1
  connections:
  A/RConn1 -- Ideal Switch/LConn1
  a/RConn1 -- Ideal Switch/RConn1
  B/RConn1 -- Ideal Switch1/LConn1
  b/RConn1 -- Ideal Switch1/RConn1
  C/RConn1 -- Ideal Switch2/LConn1
  c/RConn1 -- Ideal Switch2/RConn1

== system Teste_sem_maquina_sincrona/Secondary Distribution (circuit breakers)/Contactor1 ==
  com : Inport
  Ideal Switch : powerlib/Power Electronics/Ideal Switch  Ron=0.001  Lon=0  IC=0  Rs=1e3  Cs=inf  Measurements=off
  Ideal Switch1 : powerlib/Power Electronics/Ideal Switch  Ron=0.001  Lon=0  IC=0  Rs=1e3  Cs=inf  Measurements=off
  Ideal Switch2 : powerlib/Power Electronics/Ideal Switch  Ron=0.001  Lon=0  IC=0  Rs=1e3  Cs=inf  Measurements=off
  A : PMIOPort  Port=1  Side=Left
  a : PMIOPort  Port=2  Side=Right
  B : PMIOPort  Port=3  Side=Left
  b : PMIOPort  Port=4  Side=Right
  C : PMIOPort  Port=5  Side=Left
  c : PMIOPort  Port=6  Side=Right
  wires:
  com/1 -> Ideal Switch1/1, Ideal Switch2/1, Ideal Switch/1
  connections:
  c/RConn1 -- Ideal Switch2/RConn1
  C/RConn1 -- Ideal Switch2/LConn1
  b/RConn1 -- Ideal Switch1/RConn1
  B/RConn1 -- Ideal Switch1/LConn1
  a/RConn1 -- Ideal Switch/RConn1
  A/RConn1 -- Ideal Switch/LConn1

== system Teste_sem_maquina_sincrona/Secondary Distribution (circuit breakers)/Contactor2 ==
  com : Inport
  Ideal Switch : powerlib/Power Electronics/Ideal Switch  Ron=0.001  Lon=0  IC=0  Rs=1e3  Cs=inf  Measurements=off
  Ideal Switch1 : powerlib/Power Electronics/Ideal Switch  Ron=0.001  Lon=0  IC=0  Rs=1e3  Cs=inf  Measurements=off
  Ideal Switch2 : powerlib/Power Electronics/Ideal Switch  Ron=0.001  Lon=0  IC=0  Rs=1e3  Cs=inf  Measurements=off
  A : PMIOPort  Port=1  Side=Left
  a : PMIOPort  Port=2  Side=Right
  B : PMIOPort  Port=3  Side=Left
  b : PMIOPort  Port=4  Side=Right
  C : PMIOPort  Port=5  Side=Left
  c : PMIOPort  Port=6  Side=Right
  wires:
  com/1 -> Ideal Switch/1, Ideal Switch2/1, Ideal Switch1/1
  connections:
  A/RConn1 -- Ideal Switch/LConn1
  a/RConn1 -- Ideal Switch/RConn1
  B/RConn1 -- Ideal Switch1/LConn1
  b/RConn1 -- Ideal Switch1/RConn1
  C/RConn1 -- Ideal Switch2/LConn1
  c/RConn1 -- Ideal Switch2/RConn1

== system Teste_sem_maquina_sincrona/Secondary Distribution (circuit breakers)/Contactor3 ==
  com : Inport
  Ideal Switch : powerlib/Power Electronics/Ideal Switch  Ron=0.001  Lon=0  IC=0  Rs=1e3  Cs=inf  Measurements=off
  Ideal Switch1 : powerlib/Power Electronics/Ideal Switch  Ron=0.001  Lon=0  IC=0  Rs=1e3  Cs=inf  Measurements=off
  Ideal Switch2 : powerlib/Power Electronics/Ideal Switch  Ron=0.001  Lon=0  IC=0  Rs=1e3  Cs=inf  Measurements=off
  A : PMIOPort  Port=1  Side=Left
  a : PMIOPort  Port=2  Side=Right
  B : PMIOPort  Port=3  Side=Left
  b : PMIOPort  Port=4  Side=Right
  C : PMIOPort  Port=5  Side=Left
  c : PMIOPort  Port=6  Side=Right
  wires:
  com/1 -> Ideal Switch1/1, Ideal Switch2/1, Ideal Switch/1
  connections:
  c/RConn1 -- Ideal Switch2/RConn1
  C/RConn1 -- Ideal Switch2/LConn1
  b/RConn1 -- Ideal Switch1/RConn1
  B/RConn1 -- Ideal Switch1/LConn1
  a/RConn1 -- Ideal Switch/RConn1
  A/RConn1 -- Ideal Switch/LConn1
